simulink model "nonlinear_simulation_2017b_compare_controllers"  (R2021a)
settings: Solver=VariableStepAuto  StartTime=0.0  StopTime=500  RelTol=1e-3
StartFcn:
  | load('LTI_controller_continuous')
  | load('LTI_controller_continuous_2')
StopFcn:
  | err = out.ref.Data - out.pos.Data;
  | mse = sqrt(sum(vecnorm(err, 2).^2)) / length(err);
  | 
  | figure()
  | plot3(out.ref.Data(:,1),out.ref.Data(:,2),out.ref.Data(:,3))
  | hold on
  | plot3(out.pos.Data(:,1),out.pos.Data(:,2),out.pos.Data(:,3))
  | hold off
  | 
  | title(sprintf('MSE: %g', mse))
values from neighbouring files (symbols this model uses):
  d = 0.15    [Hinfsyn_approx_hippocampus.m]    (also in LTI_controller_continuous_2.mat; LTI_controller_continuous_3.mat)
  K2 = K    [Hinfsyn_approx_hippocampus.m]
undefined symbols (not defined in the file or in its folder): K
settings Model: Creator=ch  LastModifiedBy=adwai
settings SolverCC: AlgebraicLoopSolver=TrustRegion
settings DebuggingCC: SFMachineParentedDataDiag=warning  ArithmeticOperatorsInVariantConditions=warning
settings SFSimCC: CustomCodeUndefinedFunction=UseInterfaceOnly

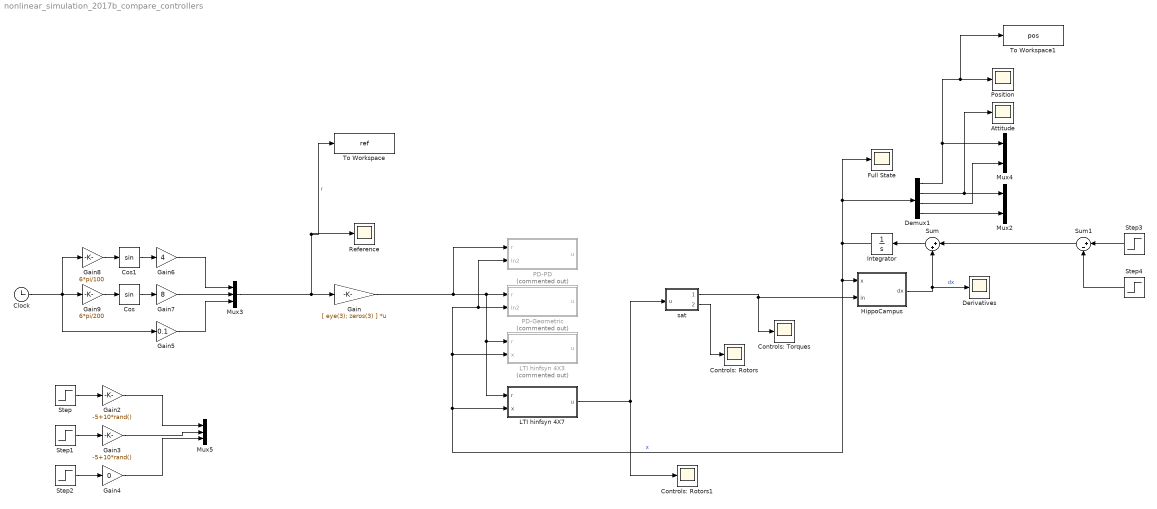
== system nonlinear_simulation_2017b_compare_controllers ==
  Attitude : Scope
  Clock : Clock
  Controls: Rotors : Scope
  Controls: Rotors1 : Scope
  Controls: Torques : Scope
  Cos : Trigonometry
  Cos1 : Trigonometry
  Demux1 : Demux  Outputs=[3 3 3 3]
  Derivatives : Scope
  Full State : Scope
  Gain : Gain  Gain=[ eye(3); zeros(3) ]  Multiplication=Matrix(K*u) (u vector)
  Gain2 : Gain  Gain=-5+10*rand()
  Gain3 : Gain  Gain=-5+10*rand()
  Gain4 : Gain  Gain=0
  Gain5 : Gain  Gain=0.1
  Gain6 : Gain  Gain=4
  Gain7 : Gain  Gain=8
  Gain8 : Gain  Gain=6*pi/100
  Gain9 : Gain  Gain=6*pi/200
  HippoCampus : MATLAB Function  TreatAsAtomicUnit=on
  Integrator : Integrator  InitialCondition=[0; 0; 0; 0;0;0;zeros(6,1)]
  LTI hinfsyn 4X3 : Subsystem  Commented=on
  LTI hinfsyn 4X7 : Subsystem
  Mux2 : Mux  Inputs=2
  Mux3 : Mux  Inputs=[1 1 1]
  Mux4 : Mux  Inputs=2
  Mux5 : Mux  Inputs=[1 1 1]
  PD-Geometric : Subsystem  Commented=on
  PD-PD : Subsystem  Commented=on
  Position : Scope
  Reference : Scope
  Step : Step  SampleTime=0
  Step1 : Step  SampleTime=0
  Step2 : Step  SampleTime=0
  Step3 : Step  Time=50  After=0.5  SampleTime=0
  Step4 : Step  Time=55  After=0.5  SampleTime=0
  Sum : Sum  Inputs=|++
  Sum1 : Sum  Inputs=|+-
  To Workspace : ToWorkspace  VariableName=ref  SaveFormat=Timeseries  SampleTime=-1
  To Workspace1 : ToWorkspace  VariableName=pos  SaveFormat=Timeseries  SampleTime=-1
  sat : MATLAB Function  TreatAsAtomicUnit=on
  wires:
  Gain9/1 -> Cos/1
  Gain6/1 -> Mux3/1
  Clock/1 -> Gain5/1, Gain9/1, Gain8/1
  Cos1/1 -> Gain6/1
  Gain8/1 -> Cos1/1
  Cos/1 -> Gain7/1
  Gain7/1 -> Mux3/2
  Gain5/1 -> Mux3/3
  HippoCampus/1(dx) -> Sum/2, Derivatives/1  "dx"
  Integrator/1 -> PD-PD/2(In2), PD-Geometric/2(In2), LTI hinfsyn 4X3/2(x), LTI hinfsyn 4X7/2(x), HippoCampus/1(x), Demux1/1, Full State/1  "x"
  Demux1/1 -> Mux4/1, To Workspace1/1, Position/1
  Demux1/2 -> Attitude/1, Mux2/1
  Demux1/4 -> Mux2/2
  Demux1/3 -> Mux4/2
  Gain/1 -> PD-PD/1(r), LTI hinfsyn 4X7/1(r), LTI hinfsyn 4X3/1(r), PD-Geometric/1(r)
  Step/1 -> Gain2/1
  Step1/1 -> Gain3/1
  Step2/1 -> Gain4/1
  Gain2/1 -> Mux5/1
  Gain3/1 -> Mux5/2
  Gain4/1 -> Mux5/3
  Sum/1 -> Integrator/1
  Step3/1 -> Sum1/1
  Step4/1 -> Sum1/2
  Sum1/1 -> Sum/1
  Mux3/1 -> To Workspace/1, Reference/1, Gain/1  "r"
  sat/1(u_sat) -> HippoCampus/2(in), Controls: Torques/1
  sat/2(omega) -> Controls: Rotors/1
  LTI hinfsyn 4X7/1(u) -> sat/1(u), Controls: Rotors1/1

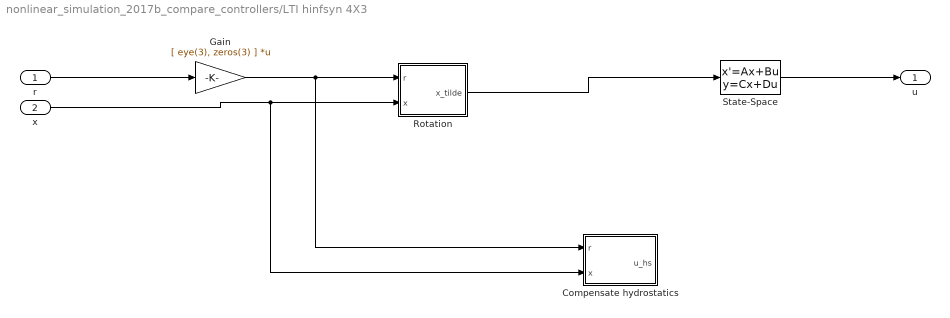
== system nonlinear_simulation_2017b_compare_controllers/LTI hinfsyn 4X3 ==
  r : Inport
  x : Inport  Port=2
  Compensate hydrostatics : MATLAB Function  TreatAsAtomicUnit=on
  Gain : Gain  Gain=[ eye(3), zeros(3) ]  Multiplication=Matrix(K*u) (u vector)
  Rotation : MATLAB Function  TreatAsAtomicUnit=on
  State-Space : StateSpace  A=K.A  B=K.B  C=K.C  D=K.D  InitialCondition=0
  u : Outport
  wires:
  State-Space/1 -> u/1
  r/1 -> Gain/1
  Gain/1 -> Compensate hydrostatics/1(r), Rotation/1(r)
  x/1 -> Compensate hydrostatics/2(x), Rotation/2(x)
  Rotation/1(x_tilde) -> State-Space/1

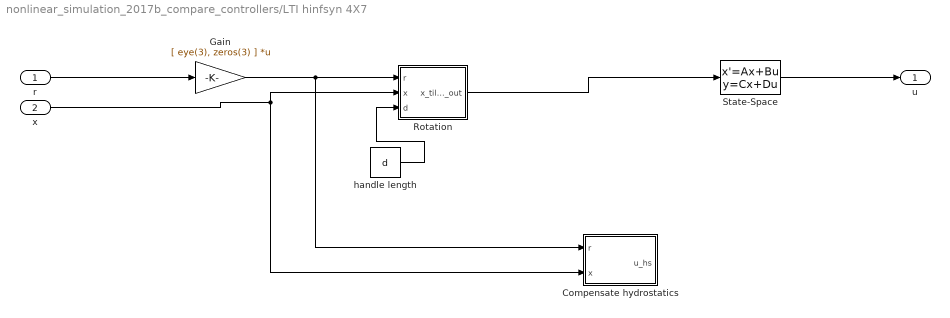
== system nonlinear_simulation_2017b_compare_controllers/LTI hinfsyn 4X7 ==
  r : Inport
  x : Inport  Port=2
  Compensate hydrostatics : MATLAB Function  TreatAsAtomicUnit=on
  Gain : Gain  Gain=[ eye(3), zeros(3) ]  Multiplication=Matrix(K*u) (u vector)
  Rotation : MATLAB Function  TreatAsAtomicUnit=on
  State-Space : StateSpace  A=K2.A  B=K2.B  C=K2.C  D=K2.D  InitialCondition=0
  handle length : Constant  Value=d
  u : Outport
  wires:
  State-Space/1 -> u/1
  r/1 -> Gain/1
  Gain/1 -> Compensate hydrostatics/1(r), Rotation/1(r)
  x/1 -> Compensate hydrostatics/2(x), Rotation/2(x)
  Rotation/1(x_tilde_out) -> State-Space/1
  handle length/1 -> Rotation/3(d)

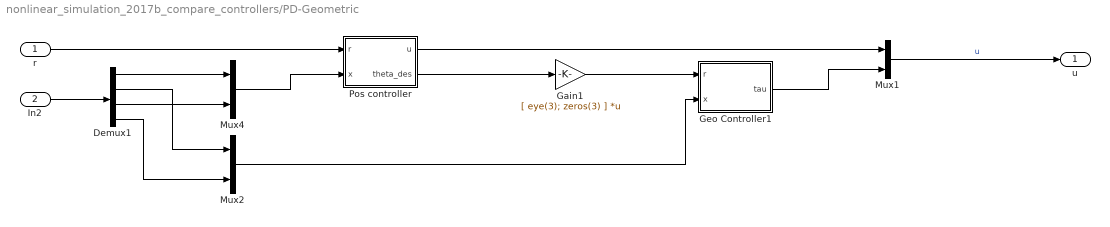
== system nonlinear_simulation_2017b_compare_controllers/PD-Geometric ==
  r : Inport
  In2 : Inport  Port=2
  Demux1 : Demux  Outputs=[3 3 3 3]
  Gain1 : Gain  Gain=[ eye(3); zeros(3) ]  Multiplication=Matrix(K*u) (u vector)
  Geo Controller1 : MATLAB Function  TreatAsAtomicUnit=on
  Mux1 : Mux  Inputs=2
  Mux2 : Mux  Inputs=2
  Mux4 : Mux  Inputs=2
  Pos controller : MATLAB Function  TreatAsAtomicUnit=on
  u : Outport
  wires:
  Geo Controller1/1(tau) -> Mux1/2
  Mux1/1 -> u/1  "u"
  Pos controller/1(u) -> Mux1/1
  r/1 -> Pos controller/1(r)
  In2/1 -> Demux1/1
  Demux1/1 -> Mux4/1
  Demux1/3 -> Mux4/2
  Mux4/1 -> Pos controller/2(x)
  Demux1/2 -> Mux2/1
  Demux1/4 -> Mux2/2
  Mux2/1 -> Geo Controller1/2(x)
  Pos controller/2(theta_des) -> Gain1/1
  Gain1/1 -> Geo Controller1/1(r)

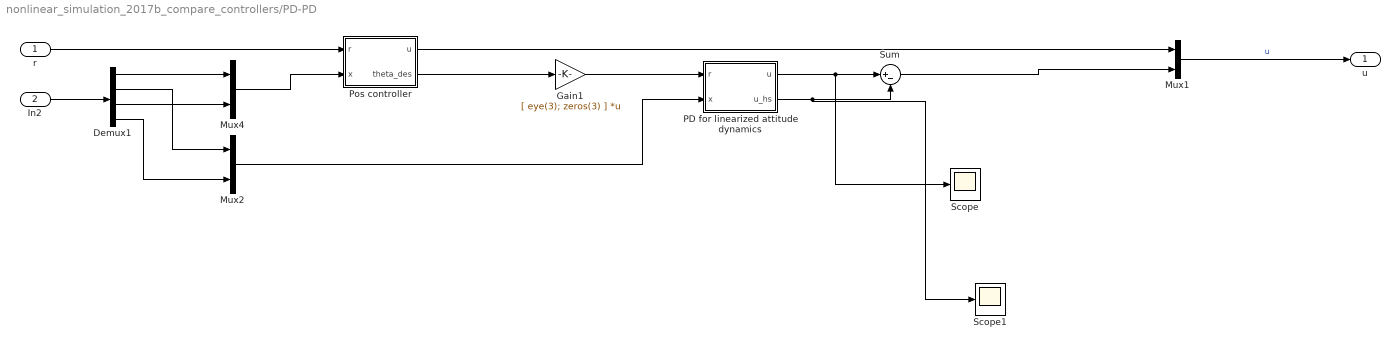
== system nonlinear_simulation_2017b_compare_controllers/PD-PD ==
  r : Inport
  In2 : Inport  Port=2
  Demux1 : Demux  Outputs=[3 3 3 3]
  Gain1 : Gain  Gain=[ eye(3); zeros(3) ]  Multiplication=Matrix(K*u) (u vector)
  Mux1 : Mux  Inputs=2
  Mux2 : Mux  Inputs=2
  Mux4 : Mux  Inputs=2
  PD for linearized attitude dynamics : MATLAB Function  TreatAsAtomicUnit=on
  Pos controller : MATLAB Function  TreatAsAtomicUnit=on
  Scope : Scope
  Scope1 : Scope
  Sum : Sum  Inputs=|+-
  u : Outport
  wires:
  Mux1/1 -> u/1  "u"
  Pos controller/1(u) -> Mux1/1
  r/1 -> Pos controller/1(r)
  In2/1 -> Demux1/1
  Demux1/1 -> Mux4/1
  Demux1/3 -> Mux4/2
  Mux4/1 -> Pos controller/2(x)
  Demux1/2 -> Mux2/1
  Demux1/4 -> Mux2/2
  Mux2/1 -> PD for linearized attitude dynamics/2(x)
  Pos controller/2(theta_des) -> Gain1/1
  Gain1/1 -> PD for linearized attitude dynamics/1(r)
  PD for linearized attitude dynamics/2(u_hs) -> Sum/2, Scope1/1
  PD for linearized attitude dynamics/1(u) -> Scope/1, Sum/1
  Sum/1 -> Mux1/2

== matlab function nonlinear_simulation_2017b_compare_controllers/PD-PD/PD for linearized attitude dynamics ==
  data: r input; x input; u output; u_hs output
function [u,u_hs] = fcn(r, x)
%% Gains
p_roll = 20;
p_pitch = 20;
p_yaw = 20;

d_roll = 3;
d_pitch = 8;
d_yaw = 8;

K_p = diag([p_roll, p_pitch, p_yaw]);
K_d = diag([d_roll, d_pitch, d_yaw]);

%% Compute control errors
u = K_p * (r(1:3)-x(1:3)) + K_d * (r(4:6)-x(4:6));

%% Remove the hydrostatic forces
zg = 0.05; % [m]
g  = 9.81; % [m/s^2]
m  = 1.43; % [kg]   

phi   = x(4);
theta = x(5);

% Compute hydrostatic load compensation
gravity = zg * g * m;
u_hs    = -[ gravity * cos(theta) * sin(phi); gravity * sin(theta); 0 ];
end

== matlab function nonlinear_simulation_2017b_compare_controllers/HippoCampus ==
  data: x input; dx output; in input
function dx = fcn(x, in)
    zg    =  0.05;    % [m]
    g     =  9.81;    % [m/s^2]

    m     =  1.43;    % [kg]
    Ix    = 0.00241; % [kgm^2]
    Iy    = 0.01072; % [kgm^2]
    Iz    = 0.01072; % [kgm^2]
    Xudot = -1.11;    % [kg]
    Yvdot = -2.80;    % [kg]
    Zwdot = -2.80;    % [kg]
    Kpdot = -0.0018;  % [kgm^2]
    Mqdot = -0.0095;  % [kgm^2]
    Nrdot = -0.0095;  % [kgm^2]
    Xu    = -4.56;    % [kg/m]
    Yv    = -17.36;   % [kg/m]
    Zw    = -17.36;   % [kg/m]
    Kp    = -0.0028;  % [kgm^2]
    Mq    = -0.0476;  % [kgm^2]
    Nr    = -0.0476;  % [kgm^2]

    % Extract states into more readable form
    phi = x( 4); theta = x( 5);
    u   = x( 7); v     = x( 8); w   = x( 9);
    p   = x(10); q     = x(11); r   = x(12);
    nu  = x(7:12);

    % Construct rotational tensor
    R = body_frame_rotation(x(4:6));

    % Construct velocity transformation tensor
    T = [ 1  sin(phi)*tan(theta)   cos(phi)*tan(theta) ;
          0  cos(phi)             -sin(phi)            ;
          0  sin(phi)/cos(theta)   cos(phi)/cos(theta) ];
    J = [ R         zeros(3) ;
          zeros(3)  T        ];

    % Calculate mass matrix
    Ma  = -diag([Xudot, Yvdot, Zwdot, Kpdot, Mqdot, Nrdot]);
    Mrb =  diag([m,  m,  m, Ix, Iy, Iz]);
    M = Ma + Mrb;

    % Compute hydrostatic load
    gravity = zg * g * m;
    G = [ 0; 0; 0; gravity * cos(theta) * sin(phi); gravity * sin(theta); 0 ];

    % Construct coriolis matrix, see Fossen 2011, Theorem 3.2
    C12 = -skew(M(1:3,1:3) * nu(1:3));
    C = [ zeros(3)   C12                        ;
          C12       -skew(M(4:6,4:6) * nu(4:6)) ];

    % Construct damping matrix
    D = -diag([Xu * abs(u), Yv * abs(v),...
               Zw * abs(w), Kp * abs(p),...
               Mq * abs(q), Nr * abs(r)]);

    % Build state space equations
    tau  = [ in(1); 0; 0; in(2:4) ];

    dx       = zeros(12,1);
    dx(1:6)  = J*nu;
    dx(7:12) = M \ (tau - (C+D)*nu - G);
end

function S = skew(lambda)
    S = [  0          -lambda(3)   lambda(2) ;
           lambda(3)   0          -lambda(1) ;
          -lambda(2)   lambda(1)   0         ]; 
end

function R = body_frame_rotation(Phi)
    phi = Phi(1); theta = Phi(2); psi = Phi(3);

    R = [  cos(psi)*cos(theta)  cos(psi)*sin(theta)*sin(phi)-sin(psi)*cos(phi)  cos(psi)*cos(phi)*sin(theta)+sin(psi)*sin(phi) ;
           sin(psi)*cos(theta)  sin(psi)*sin(theta)*sin(phi)+cos(psi)*cos(phi)  sin(psi)*cos(phi)*sin(theta)-cos(psi)*sin(phi) ;
          -sin(theta)           cos(theta)*sin(phi)                             cos(theta)*cos(phi)                            ];
end

== matlab function nonlinear_simulation_2017b_compare_controllers/LTI hinfsyn 4X3/Rotation ==
  data: r input; x_tilde output; x input
function x_tilde = fcn(r,x)
  phi = x(4);
  theta = x(5);
  psi = x(6);
  d = 0.01;
  e=r-x(1:3,1);
  R = [  cos(psi)*cos(theta)  cos(psi)*sin(theta)*sin(phi)-sin(psi)*cos(phi)  cos(psi)*cos(phi)*sin(theta)+sin(psi)*sin(phi) ;
         sin(psi)*cos(theta)  sin(psi)*sin(theta)*sin(phi)+cos(psi)*cos(phi)  sin(psi)*cos(phi)*sin(theta)-cos(psi)*sin(phi) ;
        -sin(theta)           cos(theta)*sin(phi)                             cos(theta)*cos(phi)                            ];

  x_tilde = R'*e + [d;0;0];
end

== matlab function nonlinear_simulation_2017b_compare_controllers/PD-PD/Pos controller ==
  data: r input; x input; u output; theta_des output
function [u,theta_des] = fcn(r, x)
%% Heuristic position controller
% Just wrap around a hueristic position controller around the attitude
% controller
%
k_pos=2;
k_vel=2;

e=x(1:3,1)-r(1:3,1);
v_des=-k_pos*norm(e,2);
u=k_vel*(v_des-x(4));

proj_dist_xy=norm(e(1:2,1),2);
pitch_des=-atan2(e(3,1),proj_dist_xy);
psi_des=atan2(e(2),e(1));
theta_des=[0;pitch_des;psi_des];

end

== matlab function nonlinear_simulation_2017b_compare_controllers/sat ==
  data: u input; u_sat output; omega output
function [u_sat, omega] = fcn(u)
  %  u_sat=u;
    h     = 0.0481;   % [m] Distance of rotors to HippoCampus center
    Cd    = 0.0024;   % Coefficient of drag for the rotors
    tlim  = 3;        % Maximal torque of the motors 

    Q = [1,1,1,1;-Cd,Cd,-Cd,Cd;-h,-h,h,h;h,-h,-h,h];
    Qinv = inv(Q);

    % Transform into rotor space
    omega = Qinv*u;

    % Calculate utilization of each rotor
    util  = abs(omega/tlim);

    % Saturate torque at max utilization
    omega = omega ./ max(util, 1);    

    %Transform back into body frame
   u_sat = Q * omega;   
end

== matlab function nonlinear_simulation_2017b_compare_controllers/PD-Geometric/Pos controller ==
  data: r input; x input; u output; theta_des output
function [u,theta_des] = fcn(r, x)
%% Heuristic position controller
% Just wrap around a hueristic position controller around the attitude
% controller
%
k_pos=2;
k_vel=2;

e=x(1:3,1)-r(1:3,1);
v_des=-k_pos*norm(e,2);
u=k_vel*(v_des-x(4));

proj_dist_xy=norm(e(1:2,1),2);
pitch_des=-atan2(e(3,1),proj_dist_xy);
psi_des=atan2(e(2),e(1));
theta_des=[0;pitch_des;psi_des];

end

== matlab function nonlinear_simulation_2017b_compare_controllers/PD-Geometric/Geo Controller1 ==
  data: r input; x input; tau output
function tau = fcn(r, x)
%% Geo Controller following
% D. Mellinger and V. Kumar. Minimum Snap Trajectory Generation and Control
% for Quadrotors. ICRA, 2011
% D.A. Duecker,  A. Hackbarth, T. Johannink, E. Kreuzer, and E. Solowjow. 
% Micro Underwater Vehicle Hydrobatics: A Submerged Furuta Pendulum. ICRA,
% 2018.
%

%% Gains
p_roll  = 4;
p_pitch = 4;
p_yaw   = 4;

d_roll  = 1.5;
d_pitch = 2;
d_yaw   = 2;

K_p = diag([p_roll, p_pitch, p_yaw]);
K_d = diag([d_roll, d_pitch, d_yaw]);

%% Transform attitude into SO(3)
Phi     = x(1:3);
Phi_des = r(1:3);

R       = R_euler(Phi);
R_des   = R_euler(Phi_des);

%% Compute control errors

% Compute attitude error on SO(3)
e_R = 0.5*(R_des'*R - R'*R_des);

% Extract the skew-symmetric part of the rotation error matrix as a vector
e_R_vec = [e_R(3,2); e_R(1,3); e_R(2,1)]; 

% Compute the error in the angular velocities
omega     = x(4:6);
omega_des = r(4:6);
e_omega   = omega - omega_des;

%% Compute controller output
% Apply gains given as parameters
tau = - K_p * e_R_vec - K_d * e_omega;

end

function R = R_euler(Phi)
%R_EULER Function that maps the Z-Y-X Euler angles to the corresponding
%rotation matrix

phi = Phi(1); theta = Phi(2); psi = Phi(3);

R = [  cos(psi)*cos(theta)  cos(psi)*sin(theta)*sin(phi)-sin(psi)*cos(phi)  cos(psi)*cos(phi)*sin(theta)+sin(psi)*sin(phi) ;
       sin(psi)*cos(theta)  sin(psi)*sin(theta)*sin(phi)+cos(psi)*cos(phi)  sin(psi)*cos(phi)*sin(theta)-cos(psi)*sin(phi) ;
      -sin(theta)           cos(theta)*sin(phi)                             cos(theta)*cos(phi)                            ];
end

== matlab function nonlinear_simulation_2017b_compare_controllers/LTI hinfsyn 4X3/Compensate hydrostatics ==
  data: r input; x input; u_hs output
function u_hs  = fcn(r, x)

%% Remove the hydrostatic forces

zg    =  0.05;    % [m]
    g     =  9.81;    % [m/s^2]

    m     =  1.43;    % [kg]
    Ix    = 0.00241; % [kgm^2]
    Iy    = 0.01072; % [kgm^2]
    Iz    = 0.01072; % [kgm^2]
    Xudot = -1.11;    % [kg]
    Yvdot = -2.80;    % [kg]
    Zwdot = -2.80;    % [kg]
    Kpdot = -0.0018;  % [kgm^2]
    Mqdot = -0.0095;  % [kgm^2]
    Nrdot = -0.0095;  % [kgm^2]
    Xu    = -4.56;    % [kg/m]
    Yv    = -17.36;   % [kg/m]
    Zw    = -17.36;   % [kg/m]
    Kp    = -0.0028;  % [kgm^2]
    Mq    = -0.0476;  % [kgm^2]
    Nr    = -0.0476;  % [kgm^2]
    
    
    
    phi = x( 4); theta = x( 5); psi = x( 6);
% Compute hydrostatic load
    gravity = zg * g * m;
    G = blkdiag(0,0,0, gravity * cos(theta) * (sin(phi)/(phi+eps)), gravity * (sin(theta)/(theta+eps)), 0);
 % Calculate mass matrix
    Ma  = -blkdiag(Xudot, Yvdot, Zwdot, Kpdot, Mqdot, Nrdot);
    Mrb =  blkdiag(eye(3) * m, Ix, Iy, Iz);
    M = Ma + Mrb;
    
    Mi  = inv(M);
    
u_hs=-[zeros(3),eye(3)]*G*x(1:6);
end

== matlab function nonlinear_simulation_2017b_compare_controllers/LTI hinfsyn 4X7/Compensate hydrostatics ==
  data: r input; x input; u_hs output
function u_hs  = fcn(r, x)

%% Remove the hydrostatic forces

    zg    =  0.05;    % [m]
    g     =  9.81;    % [m/s^2]
    m     =  1.43;    % [kg]
    Ix    = 0.00241; % [kgm^2]
    Iy    = 0.01072; % [kgm^2]
    Iz    = 0.01072; % [kgm^2]
    Xudot = -1.11;    % [kg]
    Yvdot = -2.80;    % [kg]
    Zwdot = -2.80;    % [kg]
    Kpdot = -0.0018;  % [kgm^2]
    Mqdot = -0.0095;  % [kgm^2]
    Nrdot = -0.0095;  % [kgm^2]
    Xu    = -4.56;    % [kg/m]
    Yv    = -17.36;   % [kg/m]
    Zw    = -17.36;   % [kg/m]
    Kp    = -0.0028;  % [kgm^2]
    Mq    = -0.0476;  % [kgm^2]
    Nr    = -0.0476;  % [kgm^2]
  
    phi = x( 4); theta = x( 5); psi = x( 6);
% Compute hydrostatic load
    gravity = zg * g * m;
    G = blkdiag(0,0,0, gravity * cos(theta) * (sin(phi)/(phi+eps)), gravity * (sin(theta)/(theta+eps)), 0);
 % Calculate mass matrix
    Ma  = -blkdiag(Xudot, Yvdot, Zwdot, Kpdot, Mqdot, Nrdot);
    Mrb =  blkdiag(eye(3) * m, Ix, Iy, Iz);
    M   = Ma + Mrb;
    
    Mi  = inv(M);
    
    u_hs=-[zeros(3),eye(3)]*G*x(1:6);
end

== matlab function nonlinear_simulation_2017b_compare_controllers/LTI hinfsyn 4X7/Rotation ==
  data: r input; x_tilde_out output; x input; d input
function x_tilde_out = fcn(r,x,d)
  phi = x(4);
  theta = x(5);
  psi = x(6);
  e=r-x(1:3,1);
  R = [  cos(psi)*cos(theta)  cos(psi)*sin(theta)*sin(phi)-sin(psi)*cos(phi)  cos(psi)*cos(phi)*sin(theta)+sin(psi)*sin(phi) ;
         sin(psi)*cos(theta)  sin(psi)*sin(theta)*sin(phi)+cos(psi)*cos(phi)  sin(psi)*cos(phi)*sin(theta)-cos(psi)*sin(phi) ;
        -sin(theta)           cos(theta)*sin(phi)                             cos(theta)*cos(phi)                            ];

  x_tilde = R'*e + [d;0;0];
  %% if the controller is  of dimension 4X7
  x_tilde_out=[x_tilde;-x(7);-x(10);-x(11);-x(12)]; % ref for the last four states is 0
end
